simulink model "CartpoleStateSpace"  (R2019b)
settings: Solver=VariableStepAuto  StartTime=0.0  StopTime=10  RelTol=1e-3  EnableMultiTasking=on
settings Model: Creator=Young  LastModifiedBy=Young
settings DataIOCC: LimitDataPoints=on  MaxDataPoints=10000
settings OptimizationCC: LifeSpan=inf
settings DebuggingCC: AllowSymbolicDim=off  SFUnexpectedBacktrackingDiag=warning  SFNoUnconditionalDefaultTransitionDiag=warning  SFExecutionAtInitializationDiag=none  ArithmeticOperatorsInVariantConditions=warning
settings SFSimCC: SimUseLocalCustomCode=off  CustomCodeUndefinedFunction=UseInterfaceOnly
settings RTWCC: RTWUseLocalCustomCode=off
settings CodeAppCC: StateflowObjectComments=on
settings GRTTargetCC: TargetLangStandard=C89/C90 (ANSI)  GeneratePreprocessorConditionals=Disable all
settings ConfigComp: CovMetricSettings=dw  CovHtmlReporting=on  CovSaveCumulativeToWorkspaceVar=on  CovSaveSingleToWorkspaceVar=on  CovExternalEMLEnable=off  CovSFcnEnable=off
settings SimscapeCC: SimscapeLogType=all  SimscapeLogSimulationStatistics=on  SimscapeLogDataHistory=10000
settings ExplorerConfigSet: InternalSimMechanicsExplorerSettings="<ExplorerConfiguration><canonicalview>planar_xy</canonicalview><AnimationSetting><BasePlaybackSpeed>1.0</BasePlaybackSpeed><PlaybackSpeedFactor>1.0</PlaybackSpeedFactor></AnimationSetting><TilePanel><TileInfo><Tiles Columns=\"1\" Count=\"1\" Rows=\"1\"><Column Weight=\"1\"/><Row Weight=\"1\"/><Tile Height=\"1\" Width=\"1\" X=\"0\" Y=\"0\"/></Tiles></TileInfo><SceneInfo><SceneViewer><BGColor><R>0.60000002384185791</R><G>0.60000002384185791</G><B>0.60000002384185791</B></BGColor><Camera><DoPerspective>off</DoPerspective><Position><X>4.00469515882129201e-08</X><Y>0.437500014369970547</Y><Z>4.13005673532405559</Z></Position><Center><X>4.00469515882129201e-08</X><Y>0.437500014369970547</Y><Z>0.0999997807353736334</Z></Center><Up><X>0</X><Y>1</Y><Z>0</Z></Up><ViewLimDist>1</ViewLimDist><YLim>2.63629057187017013</YLim><XLim>4.12000000000000011</XLim></Camera></SceneViewer></SceneInfo></TilePanel><MechEditorPanel><Cameras/><GfxPanelCameraMap/><VideoCreator><PlaybackSpeedRatio>1.0</PlaybackSpeedRatio><FrameRate>30</FrameRate><VideoFormat>Motion JPEG AVI</VideoFormat><FrameSize>auto</FrameSize></VideoCreator></MechEditorPanel></ExplorerConfiguration>"

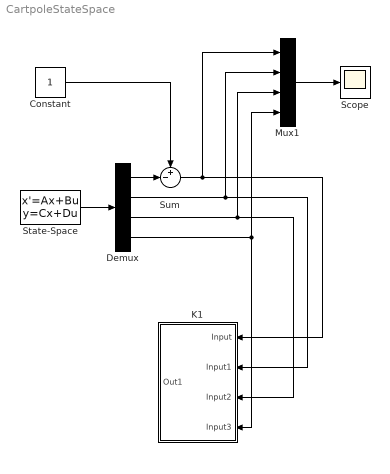
== system CartpoleStateSpace ==
  Constant : Constant
  Demux : Demux
  K1 : Subsystem  mask{K1=18.02, K2=43.26, K3=48.6, K4=11.6, PosSet=2}
      mask DialogControl ParameterGroupVar Prompt: LQR
  Mux1 : Mux
  Scope : Scope
  State-Space : StateSpace  A=[0 1 0 0;0 0 0 0;0 0 0 1;0 0 48.3 0]  B=[0;1;0;4.9]  C=[1 0 0 0;0 1 0 0;0 0 1 0;0 0 0 1]  D=[0;0;0;0]  InitialCondition=0
  Sum : Sum  Inputs=+-|
  wires:
  State-Space/1 -> Demux/1
  Demux/3 -> K1/3(Input2), Mux1/3
  Demux/4 -> K1/4(Input3), Mux1/4
  Mux1/1 -> Scope/1
  Demux/2 -> K1/2(Input1), Mux1/2
  Demux/1 -> Sum/2
  Sum/1 -> K1/1(Input), Mux1/1
  Constant/1 -> Sum/1

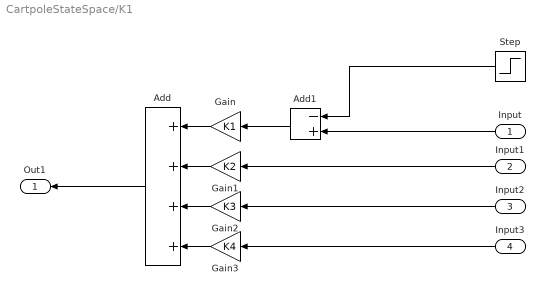
== system CartpoleStateSpace/K1 ==
  Input : Inport
  Input1 : Inport  Port=2
  Input2 : Inport  Port=3
  Input3 : Inport  Port=4
  Add : Sum  Inputs=++++
  Add1 : Sum  Inputs=-+
  Gain : Gain  Gain=K1
  Gain1 : Gain  Gain=K2
  Gain2 : Gain  Gain=K3
  Gain3 : Gain  Gain=K4
  Step : Step  After=PosSet  SampleTime=0
  Out1 : Outport
  wires:
  Gain/1 -> Add/1
  Gain1/1 -> Add/2
  Add1/1 -> Gain/1
  Gain2/1 -> Add/3
  Gain3/1 -> Add/4
  Add/1 -> Out1/1
  Step/1 -> Add1/1
  Input/1 -> Add1/2
  Input1/1 -> Gain1/1
  Input2/1 -> Gain2/1
  Input3/1 -> Gain3/1
